simulink model "Open_Lung _Model"  (R2016b)
settings: Solver=VariableStepAuto  StartTime=0.0  StopTime=10  FixedStep=0.001  RelTol=1e-3
settings Model: Creator=samiu  LastModifiedBy=Swapnil

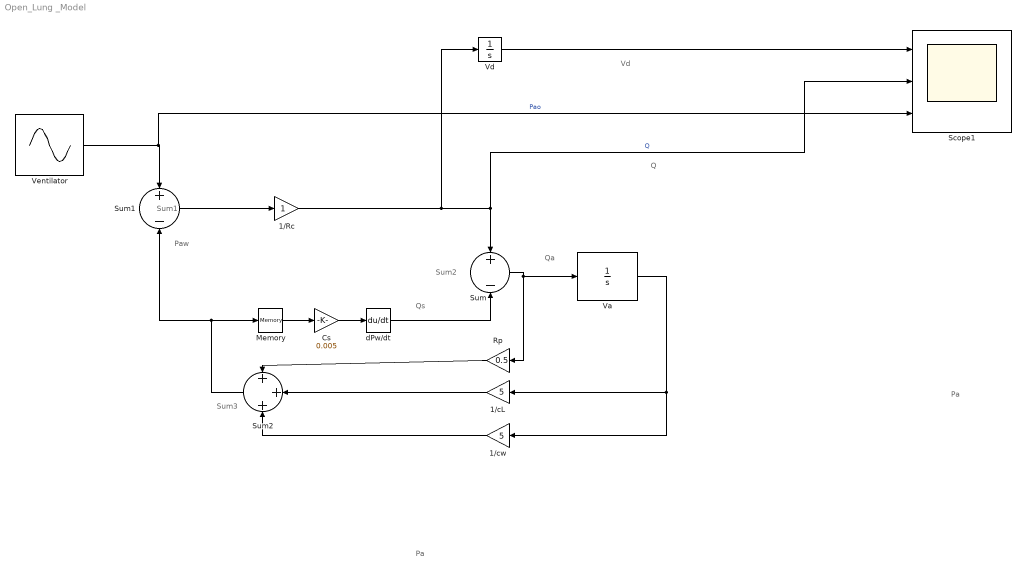
== system Open_Lung _Model ==
  note: Vd
  note: Q
  note: Pa
  note: Qs
  note: Qa
  note: Paw
  note: Sum1
  note: Sum2
  note: Sum3
  note: Pa
  1/Rc : Gain
  1/cL : Gain  Gain=5
  1/cw : Gain  Gain=5
  "Cs " : Gain  Gain=0.005
  Memory : Memory
  Rp : Gain  Gain=0.5
  Scope1 : Scope  NumInputPorts=3
  Sum : Sum  Inputs=+-
  Sum1 : Sum  Inputs=+-
  Sum2 : Sum  Inputs=+++
  Va : Integrator
  Vd : Integrator
  Ventilator : Sin  Amplitude=2.5  Frequency=1.57  SampleTime=0
  dPw/dt : Derivative
  wires:
  Ventilator/1 -> Sum1/1, Scope1/3  "Pao"
  Sum1/1 -> 1/Rc/1
  1/Rc/1 -> Vd/1, Scope1/2, Sum/1  "Q"
  Sum/1 -> Va/1, Rp/1
  Va/1 -> 1/cL/1, 1/cw/1
  Rp/1 -> Sum2/1
  1/cL/1 -> Sum2/2
  1/cw/1 -> Sum2/3
  Sum2/1 -> Sum1/2, Memory/1
  "Cs "/1 -> dPw/dt/1
  Memory/1 -> "Cs "/1
  dPw/dt/1 -> Sum/2
  Vd/1 -> Scope1/1
